simulink model "motor"  (R2024b)
settings: Solver=VariableStepAuto  StartTime=0.0  StopTime=10.0  RelTol=1e-3
undefined symbols (not defined in the file): b, J, Kd, ke, Ki, Kp, kt, L, Nf, R
settings Model: Creator=omari  LastModifiedBy=omari

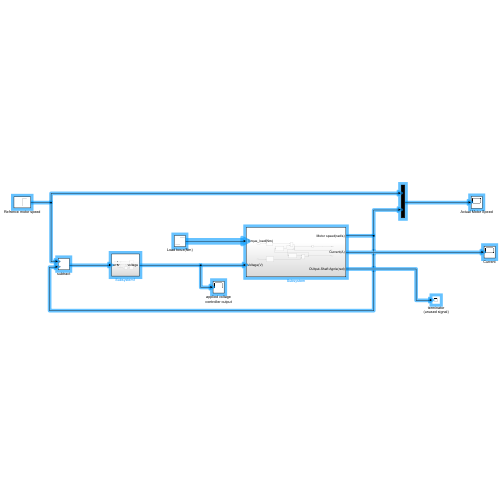
[thumbnail: Simulink's stored preview of the top-level diagram]
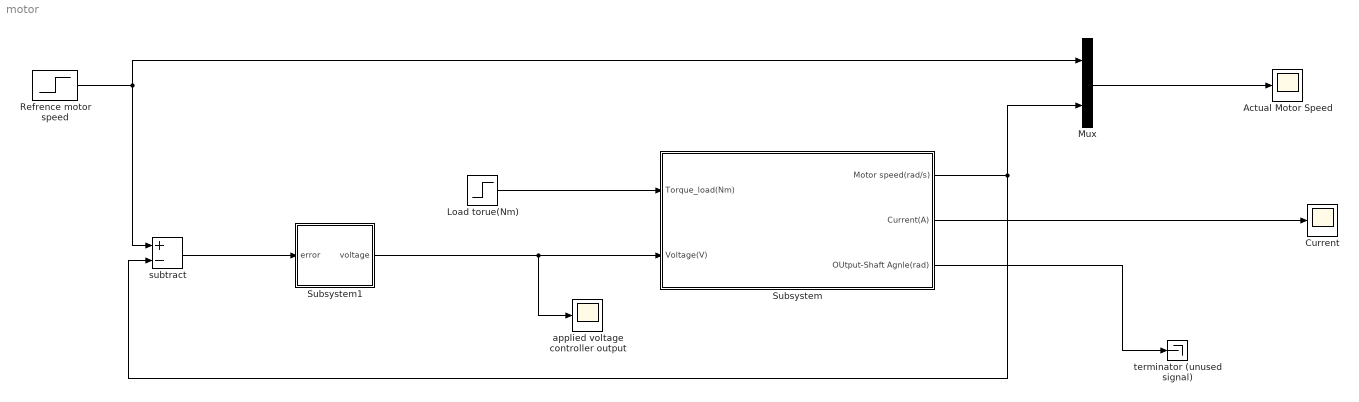
== system motor ==
  Actual Motor Speed : Scope
  Current : Scope
  Load torue(Nm) : Step  Time=15  After=0.25  SampleTime=0
  Mux : Mux  Inputs=2
  Refrence motor speed : Step  After=31.42  SampleTime=0
  Subsystem : Subsystem
  Subsystem1 : Subsystem
  applied voltage controller output : Scope
  subtract : Sum  Inputs=+-
  terminator (unused signal) : Terminator
  wires:
  Refrence motor speed/1 -> Mux/1, subtract/1
  Subsystem1/1(voltage) -> applied voltage controller output/1, Subsystem/2(Voltage(V))
  Mux/1 -> Actual Motor Speed/1
  Subsystem/2(Current(A)) -> Current/1
  Subsystem/1(Motor speed(rad/s)) -> subtract/2, Mux/2
  Subsystem/3(OUtput-Shaft Agnle(rad)) -> terminator (unused signal)/1
  subtract/1 -> Subsystem1/1(error)
  Load torue(Nm)/1 -> Subsystem/1(Torque_load(Nm))

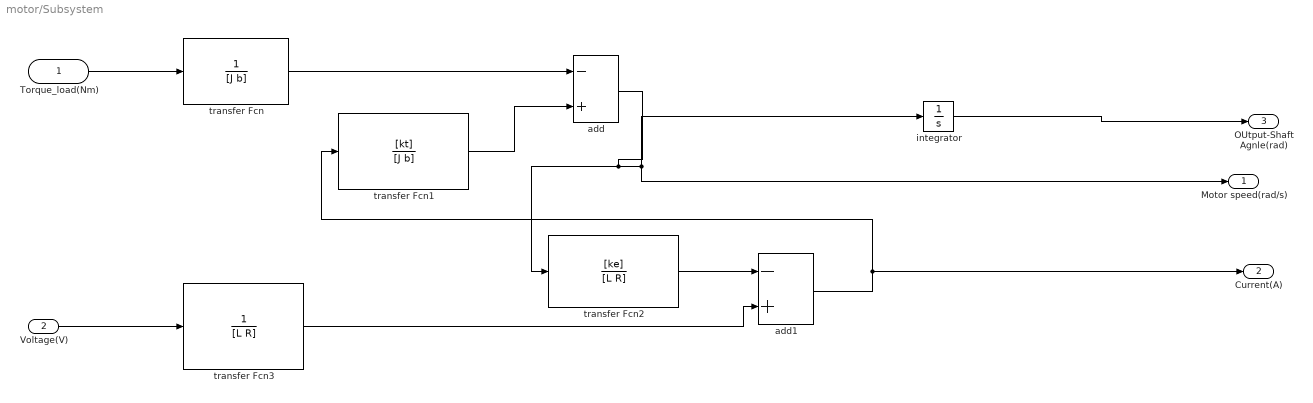
== system motor/Subsystem ==
  Torque_load(Nm) : Inport
  Voltage(V) : Inport  Port=2
  add : Sum  Inputs=-+
  add1 : Sum  Inputs=-+
  integrator : Integrator
  transfer Fcn : TransferFcn  Denominator=[J b]
  transfer Fcn1 : TransferFcn  Numerator=[kt]  Denominator=[J b]
  transfer Fcn2 : TransferFcn  Numerator=[ke]  Denominator=[L R]
  transfer Fcn3 : TransferFcn  Denominator=[L R]
  Motor speed(rad/s) : Outport
  Current(A) : Outport  Port=2
  OUtput-Shaft Agnle(rad) : Outport  Port=3
  wires:
  add/1 -> transfer Fcn2/1, Motor speed(rad/s)/1, integrator/1
  add1/1 -> Current(A)/1, transfer Fcn1/1
  Torque_load(Nm)/1 -> transfer Fcn/1
  transfer Fcn3/1 -> add1/2
  transfer Fcn2/1 -> add1/1
  Voltage(V)/1 -> transfer Fcn3/1
  transfer Fcn/1 -> add/1
  transfer Fcn1/1 -> add/2
  integrator/1 -> OUtput-Shaft Agnle(rad)/1

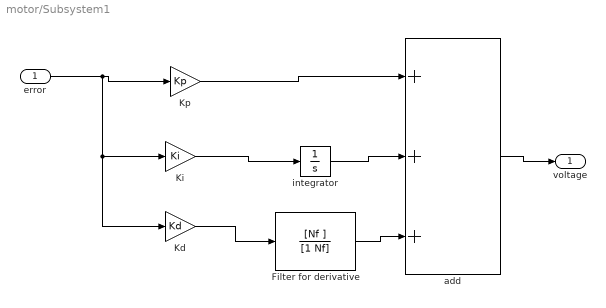
== system motor/Subsystem1 ==
  error : Inport
  Filter for derivative : TransferFcn  Numerator=[Nf ]  Denominator=[1 Nf]
  Kd : Gain  Gain=Kd
  Ki : Gain  Gain=Ki
  Kp : Gain  Gain=Kp
  add : Sum  Inputs=+++
  integrator : Integrator
  voltage : Outport
  wires:
  error/1 -> Kd/1, Ki/1, Kp/1
  Filter for derivative/1 -> add/3
  Kd/1 -> Filter for derivative/1
  Kp/1 -> add/1
  integrator/1 -> add/2
  Ki/1 -> integrator/1
  add/1 -> voltage/1
